simulink model "max_pooling_float"  (R2024b)
settings: Solver=FixedStepDiscrete  StartTime=0.0  StopTime=10.0  RelTol=1e-3
InitFcn:
  | % Define a random matrix size between 3 and 10
  | n =6;
  | 
  | fprintf('Size of matrix A: n = %d\n', n);
libraries: simulink x1
settings Model: DataTypeOverride=Off  Creator=valen  LastModifiedBy=valen
settings SolverCC: AlgebraicLoopSolver=TrustRegion
settings DataIOCC: LimitDataPoints=on  SaveOutput=off  SaveTime=off
settings OptimizationCC: BlockReduction=off  ConditionallyExecuteInputs=off  DefaultParameterBehavior=Inlined  LifeSpan=inf
settings DebuggingCC: AlgebraicLoopMsg=error  SingleTaskRateTransMsg=error  UnconnectedInputMsg=warning  UnconnectedOutputMsg=warning  UnconnectedLineMsg=warning  AllowSymbolicDim=off  StrictBusMsg=ErrorOnBusTreatedAsVector  SFUnexpectedBacktrackingDiag=warning  SFNoUnconditionalDefaultTransitionDiag=warning  SFExecutionAtInitializationDiag=none  ArithmeticOperatorsInVariantConditions=warning
settings HardwareCC: ProdBitPerPointer=32  ProdBitPerSizeT=32  ProdBitPerPtrDiffT=32  ProdLargestAtomicFloat=None  ProdIntDivRoundTo=Undefined  ProdEndianess=Unspecified  ProdWordSize=32  ProdHWDeviceType=ASIC/FPGA->ASIC/FPGA  ProdEqTarget=off
settings ModelReferenceCC: EnableRefExpFcnMdlSchedulingChecks=on
settings SFSimCC: SimUseLocalCustomCode=off  CustomCodeUndefinedFunction=UseInterfaceOnly
settings RTWCC: RTWUseLocalCustomCode=off  GPUComputeCapability=3.5
settings CodeAppCC: StateflowObjectComments=on
settings GRTTargetCC: TargetLangStandard=C89/C90 (ANSI)
settings ConfigComp: CovScope=ReferencedModels  CovMetricSettings=dw  CovSaveCumulativeToWorkspaceVar=on  CovSaveSingleToWorkspaceVar=on  CovExternalEMLEnable=off  CovSFcnEnable=off

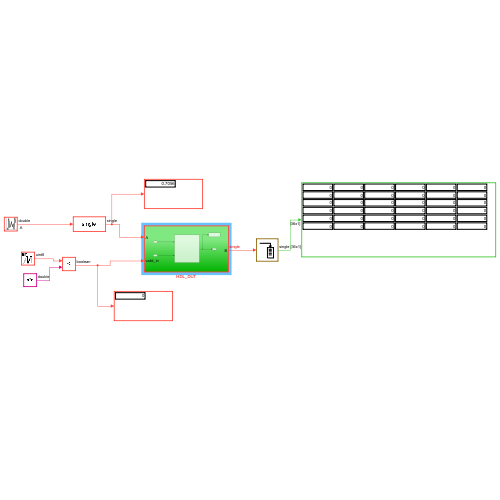
[thumbnail: Simulink's stored preview of the top-level diagram]
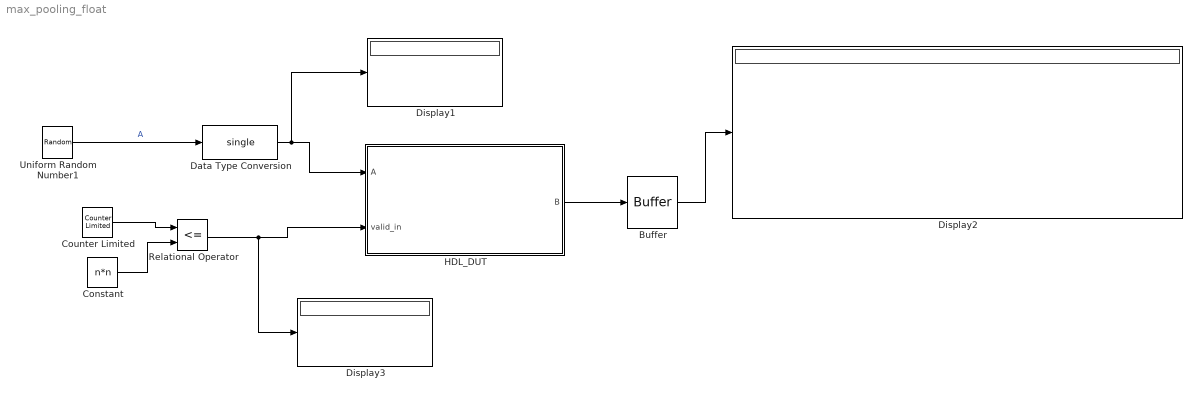
== system max_pooling_float ==
  Buffer : Buffer  N=n*n  OutputFrames=off
  Constant : Constant  Value=n*n
  Counter Limited : simulink/Sources/Counter Limited  uplimit=n*(n+1)  tsamp=-1
  Data Type Conversion : DataTypeConversion  OutDataTypeStr=single  SaturateOnIntegerOverflow=off  RndMeth=Floor
  Display1 : Display
  Display2 : Display
  Display3 : Display
  HDL_DUT : Subsystem
  Relational Operator : RelationalOperator  Operator=<=  OutDataTypeStr=boolean  RndMeth=Simplest  InputSameDT=off
  Uniform Random Number1 : UniformRandomNumber  Minimum=0  Seed=n  SampleTime=10/(n*n+1)
  wires:
  HDL_DUT/1(B) -> Buffer/1
  Constant/1 -> Relational Operator/2
  Uniform Random Number1/1 -> Data Type Conversion/1  "A"
  Counter Limited/1 -> Relational Operator/1
  Data Type Conversion/1 -> Display1/1, HDL_DUT/1(A)
  Relational Operator/1 -> Display3/1, HDL_DUT/2(valid_in)
  Buffer/1 -> Display2/1

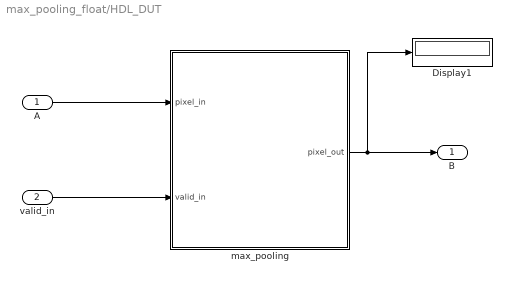
== system max_pooling_float/HDL_DUT ==
  A : Inport
  valid_in : Inport  Port=2
  Display1 : Display
  max_pooling : MATLAB Function  TreatAsAtomicUnit=on
  B : Outport  VectorParamsAs1DForOutWhenUnconnected=off
  wires:
  A/1 -> max_pooling/1(pixel_in)
  valid_in/1 -> max_pooling/2(valid_in)
  max_pooling/1(pixel_out) -> B/1, Display1/1

== matlab function max_pooling_float/HDL_DUT/max_pooling ==
  data: pixel_in input; pixel_out output; valid_in input
function pixel_out = hardware_max_pooling(pixel_in, valid_in)
    % Configuration
    SIZE = 6; 
    STRIDE = 2; 
    NUM_BLOCKS_X = SIZE / STRIDE;
    
    % Persistance des variables (Registres et RAM)
    persistent line_buffer count;
    % Lignes de retard pour aligner la latence de 3 cycles
    persistent delay_last_row delay_last_col delay_idx;
    
    if isempty(count)
        line_buffer    = zeros(1, NUM_BLOCKS_X, 'single');
        count          = int32(0);
        % Initialisation des registres de retard (taille 3 pour latence = 3)
        delay_last_row = false(1, 3);
        delay_last_col = false(1, 3);
        delay_idx      = zeros(1, 3, 'int32');
    end
    
    % Sortie par défaut
    pixel_out = single(0);
    
    if valid_in
        % 1. Détermination des coordonnées spatiales actuelles
        curr_y = floor(single(count) / SIZE);
        curr_x = mod(single(count), SIZE);
        
        % 2. Calcul de l'index du bloc horizontal actuel (1 à NUM_BLOCKS_X)
        idx_x = int32(floor(curr_x / STRIDE)) + 1;
        
        % 3. Lecture de la valeur précédemment stockée pour ce bloc
        current_max = line_buffer(idx_x);
        
        is_first_row = (mod(curr_y, STRIDE) == 0);
        is_first_col = (mod(curr_x, STRIDE) == 0);
        
        if is_first_row && is_first_col
            current_max = single(0); % Réinitialisation locale au début d'un bloc 2x2
        end
        
        % 4. Calcul du maximum cumulé (Introduit 3 cycles de latence)
        new_max = max(current_max, pixel_in);
        
        % --- GESTION DU RETARD (3 CYCLES) ---
        % On propage les signaux de contrôle dans un registre à décalage
        is_last_row_curr = (mod(curr_y, STRIDE) == (STRIDE - 1));
        is_last_col_curr = (mod(curr_x, STRIDE) == (STRIDE - 1));
        
        % Décalage (Shift Register)
        is_last_row_delayed = delay_last_row(3);
        is_last_col_delayed = delay_last_col(3);
        idx_x_delayed       = delay_idx(3);
        
        delay_last_row = [is_last_row_curr, delay_last_row(1:2)];
        delay_last_col = [is_last_col_curr, delay_last_col(1:2)];
        delay_idx      = [idx_x, delay_idx(1:2)];
        % ------------------------------------
        
        % 5. Transmission ou Stockage synchronisés (en utilisant les signaux retardés)
        if is_last_row_delayed && is_last_col_delayed
            % Fin du bloc 2x2 (3 cycles plus tard) -> On sort la valeur finale
            pixel_out = new_max;
            % On remet à zéro le buffer à l'index qui correspondait à ce pixel
            line_buffer(idx_x_delayed) = single(0);
        else
            % Au milieu du bloc 2x2 -> On sauvegarde le max temporaire au bon index
            if idx_x_delayed > 0 % Évite l'écriture au cycle 0 avant le remplissage du pipeline
                line_buffer(idx_x_delayed) = new_max;
            end
        end
                 
        % 6. Incrémentation propre du compteur de pixels
        if count >= int32((SIZE * SIZE) - 1)
            count = int32(0);
        else
            count = count + 1;
        end
    end
end
